simulink model "simulation"  (R2016a)
settings: Solver=ode45  StartTime=0.0  StopTime=100  FixedStep=0.01  MaxStep=0.01  RelTol=1e-3
values from neighbouring files (symbols this model uses):
  Adj_VL = [Adj connect'; zeros(1,N+1)]    [graph_create.m]    (also in graph_create2.m = [Adj connect; connect' 0])
  Adj_VL_2 = [Adj_2 connect2'; zeros(1,N+1)]    [graph_create.m]    (also in graph_create2.m = [Adj_2 connect_2; connect_2' 0])
  Adj_VL_2_und = adj_und(Adj_VL_2)    [main.m]
  Adj_VL_und = adj_und(Adj_VL)    [main.m]
  g = 9.81    [main.m]
  kdp = 15    [main.m]
  kdps = 15    [main.m]
  kdt = 15    [main.m]
  kdx = 1    [main.m]
  kdy = 1    [main.m]
  kdz = 20    [main.m]
  kpp = 100    [main.m]
  kpps = 100    [main.m]
  kpt = 100    [main.m]
  kpx = 1.05    [main.m]
  kpy = 1.05    [main.m]
  kpz = 100    [main.m]
  m = 0.65    [main.m]
  r_rel_1 = r_rel_but    [create_r_relative.m]
  r_rel_2 = r_rel_circle    [create_r_relative.m]
  r_rel_3 = r_rel_line    [create_r_relative.m]
  xi_init = zeros(6,N)    [main.m]
settings Model: Creator=Jens  LastModifiedBy=Jens

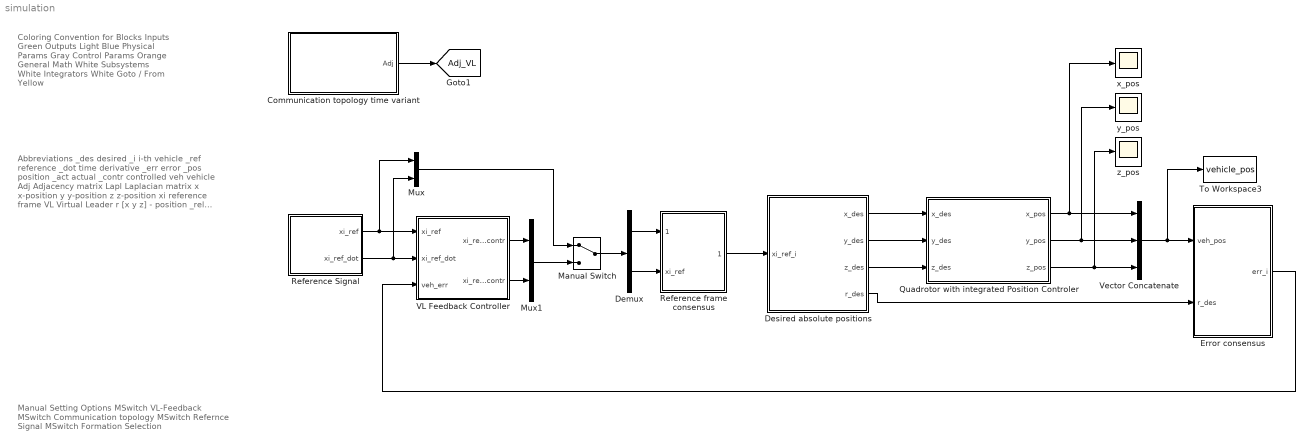
== system simulation ==
  note: Manual Setting Options
      | MSwitch VL-Feedback
      | MSwitch Communication topology
      | MSwitch Refernce Signal
      | MSwitch Formation Selection
  note: Abbreviations
      | _des desired
      | _i i-th vehicle
      | _ref reference
      | _dot time derivative
      | _err error
      | _pos position
      | _act actual
      | _contr controlled
      | veh vehicle
      | Adj Adjacency matrix
      | Lapl Laplacian matrix
      | x x-position
      | y y-position
      | z z-position
      | xi reference frame
      | VL Virtual Leader
      | r [x y z] - position
      | _rel relative in virtual frame
  note: Coloring Convention for Blocks
      | Inputs Green
      | Outputs Light Blue
      | Physical Params Gray
      | Control Params Orange
      | General Math White
      | Subsystems White
      | Integrators White
      | Goto / From Yellow
  Communication topology time variant : Subsystem
  Demux : Demux  Outputs=2
  Desired absolute positions : Subsystem
  Error consensus : Subsystem
  Manual Switch : ManualSwitch
  Mux : Mux  Inputs=2
  Mux1 : Mux  Inputs=2
  Quadrotor with integrated Position Controler : Subsystem
  Reference Signal : Subsystem
  Reference frame consensus : Subsystem
  To Workspace3 : ToWorkspace  VariableName=vehicle_pos  SaveFormat=Timeseries  SampleTime=-1
  VL Feedback Controller : Subsystem
  Vector Concatenate : Concatenate  NumInputs=3  Mode=Multidimensional array
  x_pos : Scope
  y_pos : Scope
  z_pos : Scope
  tag scope: Adj_VL=global
  wires:
  Vector Concatenate/1 -> Error consensus/1(veh_pos), To Workspace3/1
  Quadrotor with integrated Position Controler/1(x_pos) -> Vector Concatenate/1, x_pos/1
  Quadrotor with integrated Position Controler/2(y_pos) -> Vector Concatenate/2, y_pos/1
  Quadrotor with integrated Position Controler/3(z_pos) -> Vector Concatenate/3, z_pos/1
  Communication topology time variant/1(Adj) -> [Adj_VL]
  Error consensus/1(err_i) -> VL Feedback Controller/3(veh_err)
  Reference Signal/1(xi_ref) -> Mux/1, VL Feedback Controller/1(xi_ref)
  Reference Signal/2(xi_ref_dot) -> Mux/2, VL Feedback Controller/2(xi_ref_dot)
  VL Feedback Controller/1(xi_ref_dot_contr) -> Mux1/1
  VL Feedback Controller/2(xi_ref_contr) -> Mux1/2
  Mux/1 -> Manual Switch/1
  Demux/1 -> Reference frame consensus/1(xi_ref_dot)
  Demux/2 -> Reference frame consensus/2(xi_ref)
  Mux1/1 -> Manual Switch/2
  Manual Switch/1 -> Demux/1
  Reference frame consensus/1(xi_ref_i) -> Desired absolute positions/1(xi_ref_i)
  Desired absolute positions/1(x_des) -> Quadrotor with integrated Position Controler/1(x_des)
  Desired absolute positions/2(y_des) -> Quadrotor with integrated Position Controler/2(y_des)
  Desired absolute positions/3(z_des) -> Quadrotor with integrated Position Controler/3(z_des)
  Desired absolute positions/4(r_des) -> Error consensus/2(r_des)

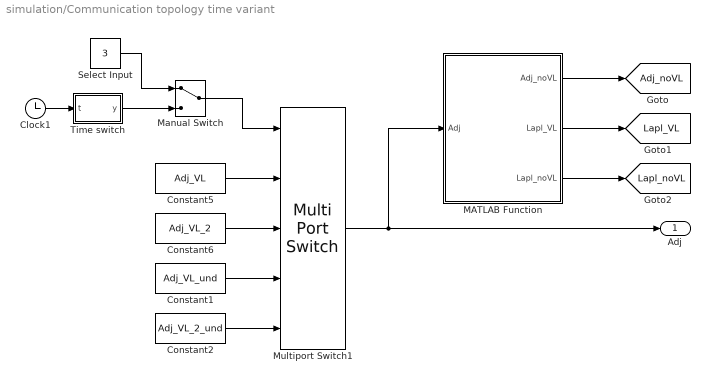
== system simulation/Communication topology time variant ==
  Clock1 : Clock
  Constant1 : Constant  Value=Adj_VL_und
  Constant2 : Constant  Value=Adj_VL_2_und
  Constant5 : Constant  Value=Adj_VL
  Constant6 : Constant  Value=Adj_VL_2
  MATLAB Function : MATLAB Function  TreatAsAtomicUnit=on
  Manual Switch : ManualSwitch
  Multiport Switch1 : MultiPortSwitch  Inputs=4
  Select Input : Constant  Value=3
  Time switch : MATLAB Function  TreatAsAtomicUnit=on
  Adj : Outport
  tag scope: Adj_noVL=global, Lapl_VL=global, Lapl_noVL=global
  wires:
  Manual Switch/1 -> Multiport Switch1/1
  Clock1/1 -> Time switch/1(t)
  Constant6/1 -> Multiport Switch1/3
  Constant5/1 -> Multiport Switch1/2
  Select Input/1 -> Manual Switch/1
  Time switch/1(y) -> Manual Switch/2
  Multiport Switch1/1 -> MATLAB Function/1(Adj), Adj/1
  Constant1/1 -> Multiport Switch1/4
  Constant2/1 -> Multiport Switch1/5
  MATLAB Function/1(Adj_noVL) -> [Adj_noVL]
  MATLAB Function/2(Lapl_VL) -> [Lapl_VL]
  MATLAB Function/3(Lapl_noVL) -> [Lapl_noVL]

== system simulation/Desired absolute positions ==
  xi_ref_i : Inport
  Desired absolute positions : MATLAB Function  TreatAsAtomicUnit=on
  To Workspace2 : ToWorkspace  VariableName=des_pos  SaveFormat=Timeseries  SampleTime=-1
  relative positions time variant : Subsystem
  x_des : Outport
  y_des : Outport  Port=2
  z_des : Outport  Port=3
  r_des : Outport  Port=4
  wires:
  Desired absolute positions/1(x_des) -> x_des/1
  Desired absolute positions/4(r_des) -> To Workspace2/1, r_des/1
  Desired absolute positions/3(z_des) -> z_des/1
  Desired absolute positions/2(y_des) -> y_des/1
  xi_ref_i/1 -> Desired absolute positions/1(xi_ref_i)
  relative positions time variant/1(r_rel_des) -> Desired absolute positions/2(r_relative)

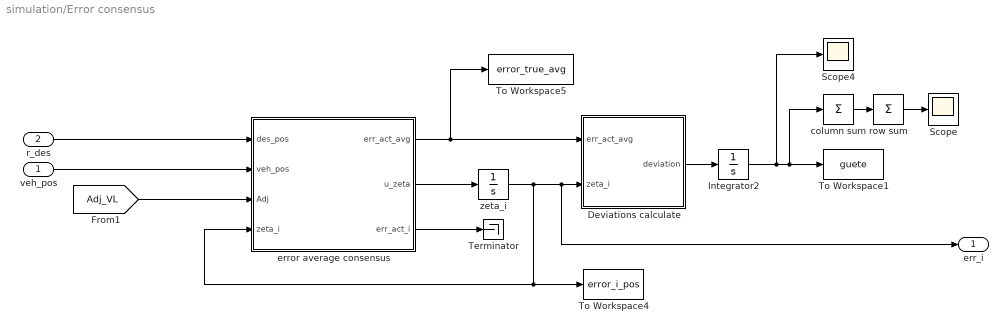
== system simulation/Error consensus ==
  veh_pos : Inport
  r_des : Inport  Port=2
  Deviations calculate : MATLAB Function  TreatAsAtomicUnit=on
  Integrator2 : Integrator
  Scope : Scope
  Scope4 : Scope
  Terminator : Terminator
  To Workspace1 : ToWorkspace  VariableName=guete  SampleTime=-1
      settings: MaxDataPoints=1
  To Workspace4 : ToWorkspace  VariableName=error_i_pos  SaveFormat=Timeseries  SampleTime=-1
  To Workspace5 : ToWorkspace  VariableName=error_true_avg  SaveFormat=Timeseries  SampleTime=-1
  column sum : Sum  Inputs=+
  error average consensus : MATLAB Function  TreatAsAtomicUnit=on
  row sum : Sum  Inputs=+
  zeta_i : Integrator
  err_i : Outport
  wires:
  r_des/1 -> error average consensus/1(des_pos)
  veh_pos/1 -> error average consensus/2(veh_pos)
  Deviations calculate/1(deviation) -> Integrator2/1
  Integrator2/1 -> column sum/1, To Workspace1/1, Scope4/1
  [Adj_VL] -> error average consensus/3(Adj)
  error average consensus/3(err_act_i) -> Terminator/1
  zeta_i/1 -> Deviations calculate/2(zeta_i), err_i/1, To Workspace4/1, error average consensus/4(zeta_i)
  error average consensus/2(u_zeta) -> zeta_i/1
  error average consensus/1(err_act_avg) -> Deviations calculate/1(err_act_avg), To Workspace5/1
  column sum/1 -> row sum/1
  row sum/1 -> Scope/1

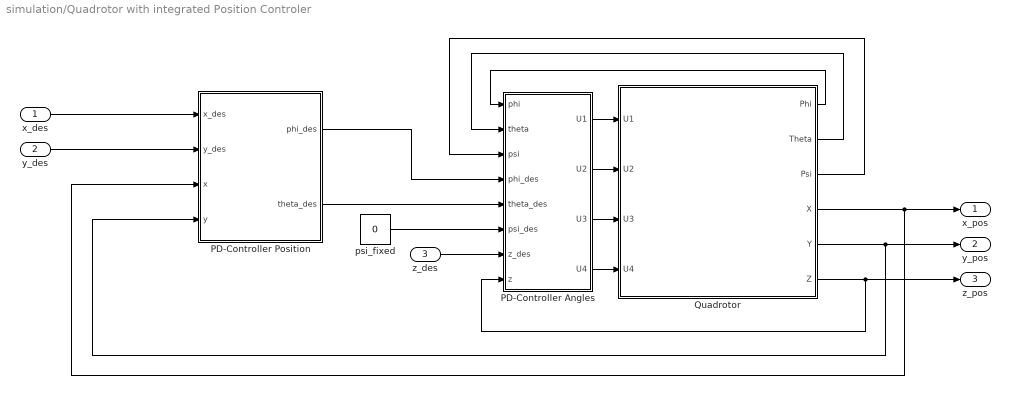
== system simulation/Quadrotor with integrated Position Controler ==
  x_des : Inport
  y_des : Inport  Port=2
  z_des : Inport  Port=3
  PD-Controller Angles : Subsystem
  PD-Controller Position : Subsystem
  Quadrotor : Subsystem
  psi_fixed : Constant  Value=0
  x_pos : Outport
  y_pos : Outport  Port=2
  z_pos : Outport  Port=3
  wires:
  PD-Controller Angles/1(U1) -> Quadrotor/1(U1)
  Quadrotor/3(Psi) -> PD-Controller Angles/3(psi)
  Quadrotor/6(Z) -> z_pos/1, PD-Controller Angles/8(z)
  PD-Controller Position/1(phi_des) -> PD-Controller Angles/4(phi_des)
  Quadrotor/2(Theta) -> PD-Controller Angles/2(theta)
  PD-Controller Position/2(theta_des) -> PD-Controller Angles/5(theta_des)
  z_des/1 -> PD-Controller Angles/7(z_des)
  Quadrotor/1(Phi) -> PD-Controller Angles/1(phi)
  PD-Controller Angles/3(U3) -> Quadrotor/3(U3)
  PD-Controller Angles/2(U2) -> Quadrotor/2(U2)
  PD-Controller Angles/4(U4) -> Quadrotor/4(U4)
  y_des/1 -> PD-Controller Position/2(y_des)
  x_des/1 -> PD-Controller Position/1(x_des)
  Quadrotor/4(X) -> x_pos/1, PD-Controller Position/3(x)
  Quadrotor/5(Y) -> y_pos/1, PD-Controller Position/4(y)
  psi_fixed/1 -> PD-Controller Angles/6(psi_des)

== system simulation/Reference Signal ==
  Integrator : Integrator  InitialCondition=[0;0;0;0;0;0]
  Mux2 : Mux  Inputs=6
  To Workspace : ToWorkspace  VariableName=xi_ref  SaveFormat=Timeseries  SampleTime=-1
  angular velocities : Subsystem
  velocities : Subsystem
  xi_ref : Outport
  xi_ref_dot : Outport  Port=2
  wires:
  Mux2/1 -> Integrator/1, xi_ref_dot/1
  Integrator/1 -> To Workspace/1, xi_ref/1
  velocities/1(x_ref_dot) -> Mux2/1
  velocities/2(y_ref_dot) -> Mux2/2
  velocities/3(z_ref_dot) -> Mux2/3
  angular velocities/1(phi_ref_dot) -> Mux2/4
  angular velocities/2(theta_ref_dot) -> Mux2/5
  angular velocities/3(psi_ref_dot) -> Mux2/6

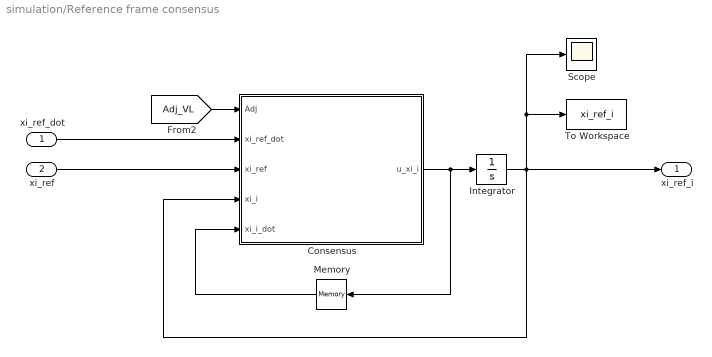
== system simulation/Reference frame consensus ==
  xi_ref_dot : Inport
  xi_ref : Inport  Port=2
  Consensus : MATLAB Function  TreatAsAtomicUnit=on
      settings: MinAlgLoopOccurrences=on
  Integrator : Integrator  InitialCondition=xi_init
  Memory : Memory
  Scope : Scope
  To Workspace : ToWorkspace  VariableName=xi_ref_i  SaveFormat=Timeseries  SampleTime=-1
  xi_ref_i : Outport
  wires:
  [Adj_VL] -> Consensus/1(Adj)
  xi_ref_dot/1 -> Consensus/2(xi_ref_dot)
  xi_ref/1 -> Consensus/3(xi_ref)
  Memory/1 -> Consensus/5(xi_i_dot)
  Consensus/1(u_xi_i) -> Integrator/1, Memory/1
  Integrator/1 -> xi_ref_i/1, To Workspace/1, Scope/1, Consensus/4(xi_i)

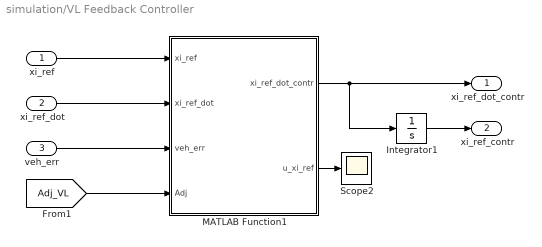
== system simulation/VL Feedback Controller ==
  xi_ref : Inport
  xi_ref_dot : Inport  Port=2
  veh_err : Inport  Port=3
  Integrator1 : Integrator
  MATLAB Function1 : MATLAB Function  TreatAsAtomicUnit=on
  Scope2 : Scope
  xi_ref_dot_contr : Outport
  xi_ref_contr : Outport  Port=2
  wires:
  MATLAB Function1/2(u_xi_ref) -> Scope2/1
  [Adj_VL] -> MATLAB Function1/4(Adj)
  xi_ref_dot/1 -> MATLAB Function1/2(xi_ref_dot)
  veh_err/1 -> MATLAB Function1/3(veh_err)
  xi_ref/1 -> MATLAB Function1/1(xi_ref)
  MATLAB Function1/1(xi_ref_dot_contr) -> Integrator1/1, xi_ref_dot_contr/1
  Integrator1/1 -> xi_ref_contr/1

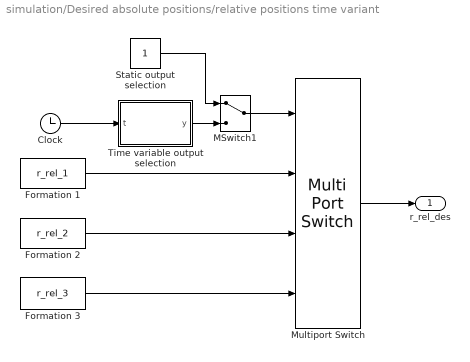
== system simulation/Desired absolute positions/relative positions time variant ==
  Clock : Clock
  Formation 1 : Constant  Value=r_rel_1
  Formation 2 : Constant  Value=r_rel_2
  Formation 3 : Constant  Value=r_rel_3
  MSwitch1 : ManualSwitch
  Multiport Switch : MultiPortSwitch
  Static output selection : Constant
  Time variable output selection : MATLAB Function  TreatAsAtomicUnit=on
  r_rel_des : Outport
  wires:
  Static output selection/1 -> MSwitch1/1
  Time variable output selection/1(y) -> MSwitch1/2
  MSwitch1/1 -> Multiport Switch/1
  Formation 1/1 -> Multiport Switch/2
  Formation 2/1 -> Multiport Switch/3
  Clock/1 -> Time variable output selection/1(t)
  Multiport Switch/1 -> r_rel_des/1
  Formation 3/1 -> Multiport Switch/4

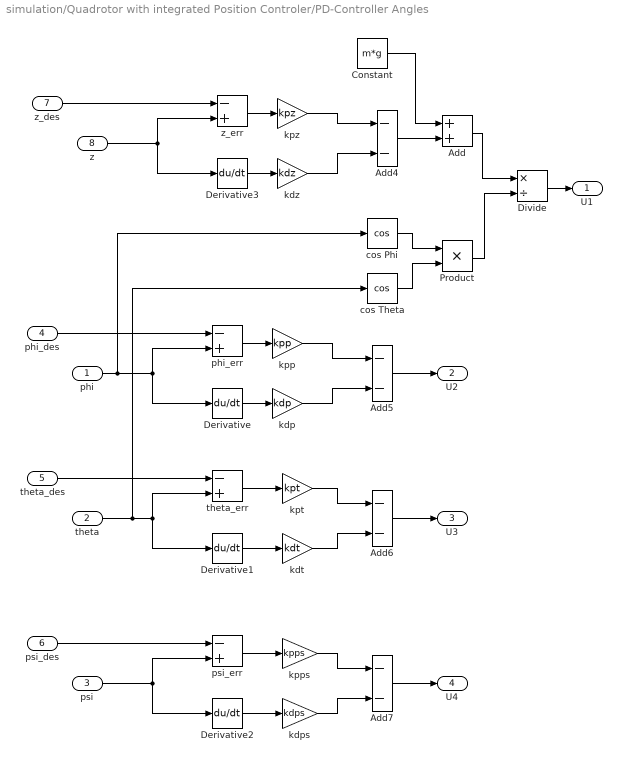
== system simulation/Quadrotor with integrated Position Controler/PD-Controller Angles ==
  phi : Inport
  theta : Inport  Port=2
  psi : Inport  Port=3
  phi_des : Inport  Port=4
  theta_des : Inport  Port=5
  psi_des : Inport  Port=6
  z_des : Inport  Port=7
  z : Inport  Port=8
  Add : Sum
  Add{4..7} (4 alike) : Sum  Inputs=--
  Constant : Constant  Value=m*g
  Derivative{,1..3} (4 alike) : Derivative
  Divide : Product  Inputs=*/
  Product : Product  RndMeth=Zero
  cos Phi : Trigonometry  Operator=cos
  cos Theta : Trigonometry  Operator=cos
  kdp : Gain  Gain=kdp
  kdps : Gain  Gain=kdps
  kdt : Gain  Gain=kdt
  kdz : Gain  Gain=kdz
  kpp : Gain  Gain=kpp
  kpps : Gain  Gain=kpps
  kpt : Gain  Gain=kpt
  kpz : Gain  Gain=kpz
  phi_err : Sum  Inputs=-+
  psi_err : Sum  Inputs=-+
  theta_err : Sum  Inputs=-+
  z_err : Sum  Inputs=-+
  U1 : Outport
  U2 : Outport  Port=2
  U3 : Outport  Port=3
  U4 : Outport  Port=4
  wires:
  phi/1 -> Derivative/1, phi_err/2, cos Phi/1
  theta/1 -> Derivative1/1, theta_err/2, cos Theta/1
  psi/1 -> Derivative2/1, psi_err/2
  phi_des/1 -> phi_err/1
  theta_des/1 -> theta_err/1
  psi_des/1 -> psi_err/1
  phi_err/1 -> kpp/1
  Derivative/1 -> kdp/1
  theta_err/1 -> kpt/1
  Derivative1/1 -> kdt/1
  psi_err/1 -> kpps/1
  Derivative2/1 -> kdps/1
  z/1 -> Derivative3/1, z_err/2
  z_des/1 -> z_err/1
  z_err/1 -> kpz/1
  Derivative3/1 -> kdz/1
  kpz/1 -> Add4/1
  kdz/1 -> Add4/2
  kpp/1 -> Add5/1
  kdp/1 -> Add5/2
  Add5/1 -> U2/1
  kpt/1 -> Add6/1
  kdt/1 -> Add6/2
  Add6/1 -> U3/1
  kpps/1 -> Add7/1
  kdps/1 -> Add7/2
  Add7/1 -> U4/1
  cos Phi/1 -> Product/1
  cos Theta/1 -> Product/2
  Add4/1 -> Add/2
  Add/1 -> Divide/1
  Product/1 -> Divide/2
  Divide/1 -> U1/1
  Constant/1 -> Add/1

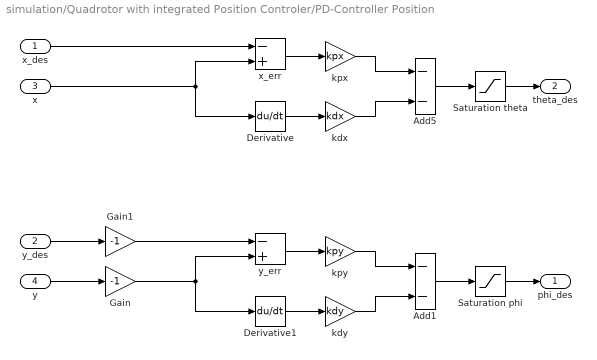
== system simulation/Quadrotor with integrated Position Controler/PD-Controller Position ==
  x_des : Inport
  y_des : Inport  Port=2
  x : Inport  Port=3
  y : Inport  Port=4
  Add1 : Sum  Inputs=--
  Add5 : Sum  Inputs=--
  Derivative : Derivative
  Derivative1 : Derivative
  Gain : Gain  Gain=-1
  Gain1 : Gain  Gain=-1
  Saturation phi : Saturate  UpperLimit=0.05  LowerLimit=-0.05  ZeroCross=off
  Saturation theta : Saturate  UpperLimit=0.05  LowerLimit=-0.05  ZeroCross=off
  kdx : Gain  Gain=kdx
  kdy : Gain  Gain=kdy
  kpx : Gain  Gain=kpx
  kpy : Gain  Gain=kpy
  x_err : Sum  Inputs=-+
  y_err : Sum  Inputs=-+
  phi_des : Outport
  theta_des : Outport  Port=2
  wires:
  x/1 -> Derivative/1, x_err/2
  x_des/1 -> x_err/1
  x_err/1 -> kpx/1
  Derivative/1 -> kdx/1
  kpx/1 -> Add5/1
  kdx/1 -> Add5/2
  Add5/1 -> Saturation theta/1
  Gain/1 -> Derivative1/1, y_err/2
  y_err/1 -> kpy/1
  Derivative1/1 -> kdy/1
  kpy/1 -> Add1/1
  kdy/1 -> Add1/2
  Add1/1 -> Saturation phi/1
  Saturation phi/1 -> phi_des/1
  y/1 -> Gain/1
  Saturation theta/1 -> theta_des/1
  y_des/1 -> Gain1/1
  Gain1/1 -> y_err/1

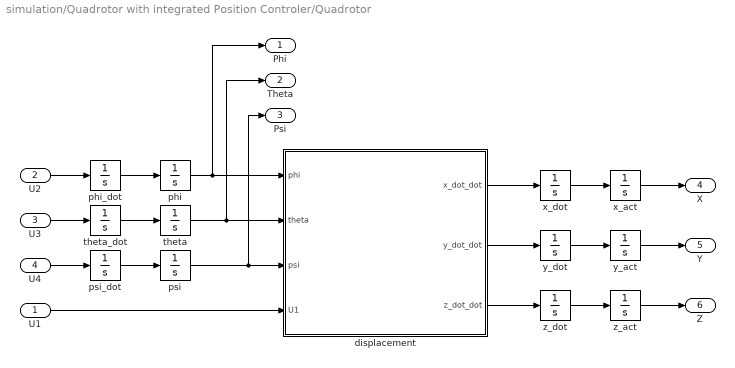
== system simulation/Quadrotor with integrated Position Controler/Quadrotor ==
  U1 : Inport
  U2 : Inport  Port=2
  U3 : Inport  Port=3
  U4 : Inport  Port=4
  displacement : Subsystem
  phi : Integrator  ZeroCross=off
  phi_dot : Integrator
  psi : Integrator  ZeroCross=off
  psi_dot : Integrator  ZeroCross=off
  theta : Integrator  ZeroCross=off
  theta_dot : Integrator  ZeroCross=off
  x_act : Integrator
  x_dot : Integrator
  y_act : Integrator
  y_dot : Integrator
  z_act : Integrator
  z_dot : Integrator
  Phi : Outport
  Theta : Outport  Port=2
  Psi : Outport  Port=3
  X : Outport  Port=4
  Y : Outport  Port=5
  Z : Outport  Port=6
  wires:
  U2/1 -> phi_dot/1
  U3/1 -> theta_dot/1
  U4/1 -> psi_dot/1
  phi_dot/1 -> phi/1
  theta_dot/1 -> theta/1
  psi_dot/1 -> psi/1
  phi/1 -> displacement/1(phi), Phi/1
  theta/1 -> displacement/2(theta), Theta/1
  psi/1 -> Psi/1, displacement/3(psi)
  displacement/1(x_dot_dot) -> x_dot/1
  x_dot/1 -> x_act/1
  y_dot/1 -> y_act/1
  displacement/2(y_dot_dot) -> y_dot/1
  z_dot/1 -> z_act/1
  displacement/3(z_dot_dot) -> z_dot/1
  x_act/1 -> X/1
  y_act/1 -> Y/1
  z_act/1 -> Z/1
  U1/1 -> displacement/4(U1)

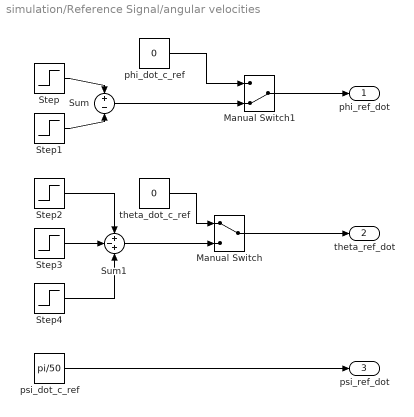
== system simulation/Reference Signal/angular velocities ==
  Manual Switch : ManualSwitch
  Manual Switch1 : ManualSwitch  CurrentSetting=0
  Step : Step  Time=20  After=pi/10  SampleTime=0
  Step1 : Step  Time=40  After=pi/10  SampleTime=0
  Step2 : Step  Time=10  After=pi/30  SampleTime=0
  Step3 : Step  Time=15  After=pi/30*2  SampleTime=0
  Step4 : Step  Time=20  After=pi/30  SampleTime=0
  Sum : Sum  Inputs=+-
  Sum1 : Sum  Inputs=+-+
  phi_dot_c_ref : Constant  Value=0
  psi_dot_c_ref : Constant  Value=pi/50
  theta_dot_c_ref : Constant  Value=0
  phi_ref_dot : Outport
  theta_ref_dot : Outport  Port=2
  psi_ref_dot : Outport  Port=3
  wires:
  Sum/1 -> Manual Switch1/2
  psi_dot_c_ref/1 -> psi_ref_dot/1
  Step1/1 -> Sum/2
  Step2/1 -> Sum1/1
  phi_dot_c_ref/1 -> Manual Switch1/1
  Manual Switch/1 -> theta_ref_dot/1
  theta_dot_c_ref/1 -> Manual Switch/1
  Step3/1 -> Sum1/2
  Step4/1 -> Sum1/3
  Manual Switch1/1 -> phi_ref_dot/1
  Step/1 -> Sum/1
  Sum1/1 -> Manual Switch/2

== system simulation/Reference Signal/velocities ==
  x_dot_c_ref = v_c_ref*cos(theta_c_ref) : Sin  Amplitude=9*pi/500  Frequency=pi/50  Phase=pi/2  SampleTime=0
  y_dot_c_ref = v_c_ref_sin(thete_c_ref) : Sin  Amplitude=9*pi/500  Frequency=pi/50  SampleTime=0
  z_dot_c_ref : Constant  Value=1/40
  x_ref_dot : Outport
  y_ref_dot : Outport  Port=2
  z_ref_dot : Outport  Port=3
  wires:
  z_dot_c_ref/1 -> z_ref_dot/1
  x_dot_c_ref = v_c_ref*cos(theta_c_ref)/1 -> x_ref_dot/1
  y_dot_c_ref = v_c_ref_sin(thete_c_ref)/1 -> y_ref_dot/1

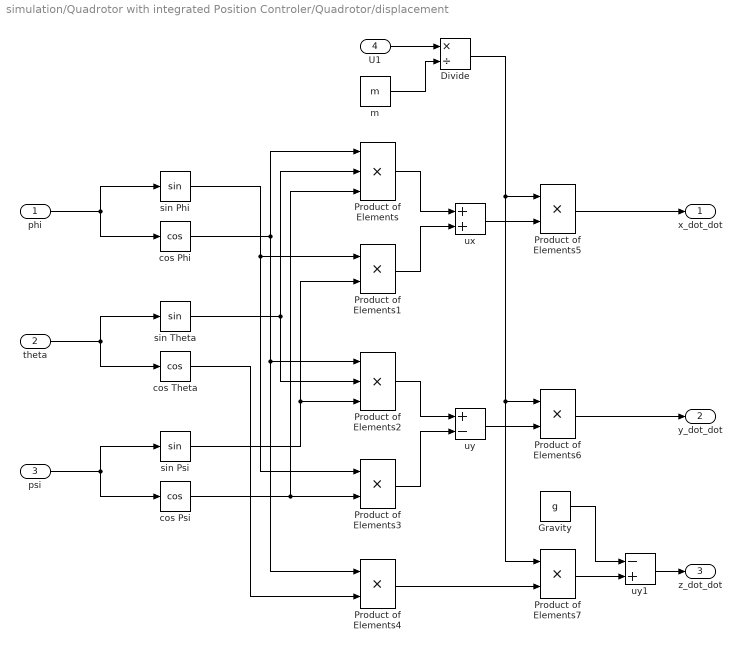
== system simulation/Quadrotor with integrated Position Controler/Quadrotor/displacement ==
  phi : Inport
  theta : Inport  Port=2
  psi : Inport  Port=3
  U1 : Inport  Port=4
  Divide : Product  Inputs=*/
  Gravity : Constant  Value=g
  Product of Elements : Product  Inputs=3
  Product of Elements{1,3..7} (6 alike) : Product
  Product of Elements2 : Product  Inputs=3
  cos Phi : Trigonometry  Operator=cos
  cos Psi : Trigonometry  Operator=cos
  cos Theta : Trigonometry  Operator=cos
  m : Constant  Value=m
  sin Phi : Trigonometry
  sin Psi : Trigonometry
  sin Theta : Trigonometry
  ux : Sum
  uy : Sum  Inputs=+-
  uy1 : Sum  Inputs=-+
  x_dot_dot : Outport
  y_dot_dot : Outport  Port=2
  z_dot_dot : Outport  Port=3
  wires:
  phi/1 -> sin Phi/1, cos Phi/1
  theta/1 -> sin Theta/1, cos Theta/1
  psi/1 -> sin Psi/1, cos Psi/1
  sin Theta/1 -> Product of Elements/2, Product of Elements2/2
  cos Psi/1 -> Product of Elements/3, Product of Elements3/2
  cos Phi/1 -> Product of Elements/1, Product of Elements2/1, Product of Elements4/1
  sin Phi/1 -> Product of Elements1/1, Product of Elements3/1
  sin Psi/1 -> Product of Elements1/2, Product of Elements2/3
  Product of Elements/1 -> ux/1
  Product of Elements1/1 -> ux/2
  ux/1 -> Product of Elements5/2
  Product of Elements2/1 -> uy/1
  Product of Elements3/1 -> uy/2
  uy/1 -> Product of Elements6/2
  cos Theta/1 -> Product of Elements4/2
  Product of Elements4/1 -> Product of Elements7/2
  U1/1 -> Divide/1
  m/1 -> Divide/2
  Divide/1 -> Product of Elements5/1, Product of Elements6/1, Product of Elements7/1
  Product of Elements5/1 -> x_dot_dot/1
  Product of Elements6/1 -> y_dot_dot/1
  uy1/1 -> z_dot_dot/1
  Product of Elements7/1 -> uy1/2
  Gravity/1 -> uy1/1

== matlab function simulation/Communication topology time variant/Time switch ==
  data: t input; y output
function y = time_switch(t)
%gives time varying output for multiport switch

if (t >= 20 && t < 60)
    y = 2;
else
    y = 1;
end

== matlab function simulation/Reference frame consensus/Consensus ==
  data: Adj input; u_xi_i output; xi_ref_dot input; xi_ref input; xi_i input; xi_i_dot input
function u_xi_i = consensus_xi(Adj, xi_ref_dot, xi_ref, xi_i, xi_i_dot)
%CONSENSUS_XI calculates u_xi = xi_i_dot for all vehicles according to the consensus
%formula for time-varying reference state (access to the leader only to a subgroup)
% Inputs:
%       Adj         - adjacency matrix
%       xi_ref_dot  - time derivative of the reference xi
%       xi_ref      - reference xi
%       xi_i        - vehicle i own understanding of reference frame
%       xi_i_dot    - vehicles i own understanding of the time derivative of xi
% Outputs:
%       u_xi_i       - control input of the i-th reference frame

% Number of vehicles
N = size(Adj,1)-1;
% initialize output u_xi to zero
u_xi_i = zeros(6,N);

% scalar to influence convergence speed
gamma = 1;

% formula to calculate xi_dot_i = u_i for each vehicle compare to thesis
% u consists of six states per vehicle in a 6xN matrix / updates each
% vehicle after another (6 states per iteration of outer for loop)
for i=1:1:N
    eta = sum(Adj(i,:));
    % if vehicle has no incoming connection (equal to eta = 0) u is set to zero therefore the
    % information states don't change and remain constant
    if (eta == 0)
        u_xi_i(:,i) = zeros(6,1);
    else
        temp = zeros(6,1);
        for j=1:1:N
            temp = temp + Adj(i,j)*(xi_i_dot(:,j)-gamma*(xi_i(:,i)-xi_i(:,j)));
        end
        u_xi_i(:,i) = 1/eta * temp + 1/eta * Adj(i,N+1)*(xi_ref_dot-gamma*(xi_i(:,i)-xi_ref));
    end    
end

== matlab function simulation/Desired absolute positions/relative positions time variant/Time variable output selection ==
  data: t input; y output
function y = fcn(t)
%gives time-varying integer output for a multiport switch

if (t < 20)
    y = 1;
elseif (t >= 20 && t < 50)
    y = 2;
elseif (t >= 50 && t < 100)
    y = 3;
else
    y = 1;
end

== matlab function simulation/Desired absolute positions/Desired absolute positions ==
  data: xi_ref_i input; x_des output; r_relative input; y_des output; z_des output; r_des output
function [x_des,y_des,z_des,r_des]  = desired_pos_abs(xi_ref_i, r_relative)
%DESIRED_POS_ABS computes the desired absolute positions depending on the
%reference frame of the vehicle and the relative coordinates of the desired
%formation (three dimensional coordinate transformation)
%
% Inputs:
%       xi_ref_i    - reference frame of the i-th vehicle
%       r_relative  - vehicle formation shape in the reference frame
% Outputs:
%       x_des       - desired x-position of the vehicle
%       y_des       - desired y-position of the vehicle
%       z_des       - desired z-position of the vehicle
%       r_relative  - combination of x,y,z-position in a matrix for all veh

% set matrix nxn
r_des = zeros(size(r_relative));

%loop over each vehicle
for i=1:1:size(r_relative,2)
    
    % information state of the vehicle angle
    psi = xi_ref_i(6,i);
    phi = xi_ref_i(5,i);
    theta = xi_ref_i(4,i);
    
    % rotational matrix Rz
    Dz = [cos(psi) -sin(psi) 0
        sin(psi)  cos(psi) 0
        0   0    1];
    
    % rotational matrix Ry
    Dy = [cos(phi)  0   sin(phi)
        0      1      0
        -sin(phi)  0   cos(phi)];
    
    % rotational matrix Rx
    Dx = [1     0         0
        0  cos(theta) -sin(theta)
        0  sin(theta)  cos(theta)];
     
    r_des(:,i) = xi_ref_i(1:3,i) + Dz*Dy*Dx*r_relative(:,i);
end

x_des = r_des(1,:);
y_des = r_des(2,:);
z_des = r_des(3,:);

end

== matlab function simulation/Error consensus/error average consensus ==
  data: des_pos input; err_act_avg output; veh_pos input; Adj input; zeta_i input; u_zeta output; err_act_i output
function [err_act_avg, u_zeta, err_act_i] = consensus_err_calc(des_pos, veh_pos, Adj, zeta_i)
%CONSENSUS_ERR_CALC computes the each vehicles own average error understanding in the formation
%it uses his own error as well as consensus to reach a good estimate of the
%average error in the network
% 
% Inputs:
%       des_pos     - desired position for each vehicle
%       veh_pos     - actual vehicle position
%       Adj         - adjacency matrix representing communication network
%       zeta_i      - information error state of each vehicle
% Outputs:
%       err_mean_act - actual mean error of all vehicles
%       u_zeta       - control input for the error state zeta
%       err_act_i    - actual error of each vehicle

beta = 20;      % scalar to set influence consensus speed
alpha = 3;      % scalar to set influence own error

% Number of vehicles
N = size(Adj,1)-1;

% true squared error in a 3xN Matrix (x,y,z) in cm
err_act_i = (100*(des_pos-veh_pos)).^2;

% initialize output u_zeta to zero
u_zeta = zeros(3,N);

% formula to calculate zeta_dot = u_zeta for each vehicle according to
% thesis formula
% u_zeta consists of three error states per vehicle in a 3xN matrix / updates each
% vehicle after another (3 states per iteration of outer for loop)
% with consensus is vehicle updating its own error into the error state
for i=1:1:N
    eta = sum(Adj(i,1:N));
    if (eta == 0)
        u_zeta(:,i) = zeros(3,1);
    else
        temp = zeros(3,1);
        for j=1:1:N
            temp = temp + Adj(i,j)*(zeta_i(:,i) - zeta_i(:,j));
        end
        % neighbor influence plus influence of own error.
        u_zeta(:,i) = -(1/eta*beta*temp + alpha*(zeta_i(:,i)-err_act_i(:,i)));
    end 
end
err_act_avg = mean(err_act_i,2);

== matlab function simulation/Error consensus/Deviations calculate ==
  data: err_act_avg input; deviation output; zeta_i input
function deviation  = dev_calc(err_act_avg, zeta_i)
%computes the deviations between the real avg error und error estimate of each vehicle
%expands the avg error to match the size of the err_i matrix
% 
% Inputs:
%       err_act_avg - actual average error in the network
% Outputs:
%       zeta_i      - average estimate of each vehicle

% number of vehicles
N = size(zeta_i,2);
deviation = abs(err_act_avg*ones(1,N)-zeta_i);

== matlab function simulation/VL Feedback Controller/MATLAB Function1 ==
  data: xi_ref_dot_contr output; xi_ref input; xi_ref_dot input; veh_err input; Adj input; u_xi_ref output
function [xi_ref_dot_contr, u_xi_ref]  = xi_ref_contr(xi_ref, xi_ref_dot, veh_err, Adj)
%XI_REF_CONTR is the controller for the reference frame xi depending on the
%average error in the network
%
% Inputs:
%       xi_ref        - reference value of the reference frame
%       xi_ref_dot    - time derivative of the reference frame

err = zeros(3,1);
N = size(Adj,1)-1;
for i=1:1:N
    if (Adj(i,N+1)==1)
        err = err + veh_err(:,i);
    end
end
err = err / sum(Adj(:,N+1));
a = 25;
b = 0.5;
u_xi_ref = 0.5*(1-(2*atan(b*(err-a)))/pi);


xi_ref_dot_contr = xi_ref_dot;
% influence of the error to the development of the reference state
xi_ref_dot_contr(1:3) = u_xi_ref.*xi_ref_dot(1:3);

== matlab function simulation/Communication topology time variant/MATLAB Function ==
  data: Adj input; Adj_noVL output; Lapl_VL output; Lapl_noVL output
function [Adj_noVL, Lapl_VL, Lapl_noVL] = lapl_adj_options(Adj)
%gives adjacency and laplacian matrix of graph with and without VL

% number of vehicles
N = size(Adj,1)-1;

% takes away last row and column
Adj_noVL = Adj(1:N,1:N);

% laplacian calculation after thesis definition
Lapl_VL = zeros(size(Adj));

for i=1:1:N+1
    for j=1:1:N+1
        if (i == j)
            % sets l(i,j) to the sum of the row without the diagonal
            % element
            Lapl_VL(i,j) = sum(Adj(i,:))-Adj(i,j);
        else
            Lapl_VL(i,j) = -Adj(i,j);
        end
    end
end
Lapl_noVL = Lapl_VL(1:N,1:N);
